simulink model "LinearControl3"  (R2019b)
settings: Solver=VariableStepAuto  StartTime=0.0  StopTime=10.0  RelTol=1e-3
settings Model: Creator=IwiLL  LastModifiedBy=IwiLL

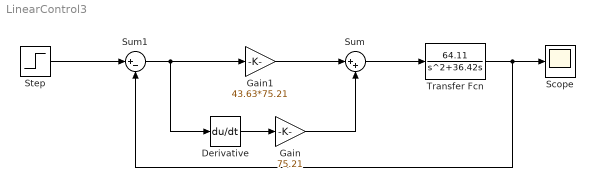
== system LinearControl3 ==
  Derivative : Derivative
  Gain : Gain  Gain=75.21
  Gain1 : Gain  Gain=43.63*75.21
  Scope : Scope
  Step : Step  Time=0  SampleTime=0
  Sum : Sum  Inputs=|++
  Sum1 : Sum  Inputs=|+-
  Transfer Fcn : TransferFcn  Numerator=[64.11]  Denominator=[1 36.42 0]
  wires:
  Step/1 -> Sum1/1
  Sum1/1 -> Derivative/1, Gain1/1
  Derivative/1 -> Gain/1
  Gain1/1 -> Sum/1
  Gain/1 -> Sum/2
  Sum/1 -> Transfer Fcn/1
  Transfer Fcn/1 -> Sum1/2, Scope/1
